simulink model "EarlyReturn20_2018a"  (R2018a)
settings: Solver=VariableStepAuto  StartTime=0.0  StopTime=0.1  RelTol=1e-3
settings Model: Creator=BEAR  LastModifiedBy=apple

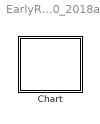
== system EarlyReturn20_2018a ==
  Chart : Stateflow chart  TreatAsAtomicUnit=on

== stateflow chart EarlyReturn20_2018a/Chart ==
  settings: updateMethod=DISCRETE  sampleTime=0.1
  state S
    en: fprintf("enS")
    du: fprintf("duS")
    ex: fprintf("exS")
    state A1
    state A2
    (junction 15) -> A2 : {fprintf("ca2")}/{fprintf("ta2")}
    A1 -> (junction 15) : {fprintf("ca1")}/{E;fprintf("ta1")}
    (default) -> A1
  state T
    en: fprintf("enT")
  (default) -> S
  S -> T : E
  events: E local FUNCTION_CALL_EVENT
